simulink model "image_view"  (Simulink 7.8)
settings: Solver=ode45  StartTime=0.0  StopTime=30.0  RelTol=1e-3
undefined symbols (not defined in the file): gray, none, videoinput
libraries: imaqlib x1, visionsinks x1
settings Model: Creator=wildcat  LastModifiedBy=wildcat

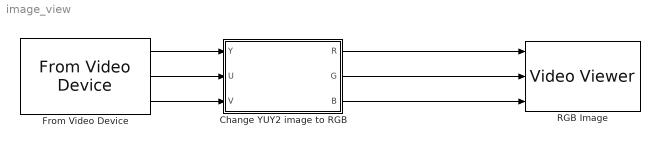
== system image_view ==
  Change YUY2 image to RGB : MATLAB Function  TreatAsAtomicUnit=on
  From Video Device : imaqlib/From Video Device  DeviceMenu=winvideo 1 (Microsoft LifeCam HD-3000)  Device=winvideo 1 (Microsoft LifeCam HD-3000)  ObjConstructor=videoinput('winvideo', 1)  VideoFormatMenu=YUY2_1280x720  VideoFormat=YUY2_1280x720  VideoSource=input1  ROIPosition=[0 0 720 1280]  EnableHWTrigger=off  TriggerConfiguration=none/none  SampleTime=1/30  OutputPortsMode=Separate color signals  DataType=uint8  CanDoHWTrigger=no  ReturnedColorSpace=YCbCr  BlockHandle=55.0015  ROIWidth=1280  ROIHeight=720  ROIColumn=0  ROIRow=0  EngXMLPath=C:\Program Files\MatlabR2011b\toolbox\imaq\imaq\private  DevXMLPath=C:\Program Files\MatlabR2011b\toolbox\imaq\imaqadaptors\win64  EngLibPath=C:\Program Files\MatlabR2011b\toolbox\imaq\imaqblks\imaqmex\win64
  RGB Image : visionsinks/Video Viewer  inputType=Obsolete7b  imagePorts=Separate color signals  useColorMap=off  colormapValue=gray(256)  specRange=off  minInputVal=0  maxInputVal=255  FigPos=[52 664 655 508]  AxisZoom=on  trueSizedOnce=off  OpenAtMdlStart=on
  wires:
  From Video Device/1 -> Change YUY2 image to RGB/1(Y)
  From Video Device/2 -> Change YUY2 image to RGB/2(U)
  From Video Device/3 -> Change YUY2 image to RGB/3(V)
  Change YUY2 image to RGB/3(B) -> RGB Image/3
  Change YUY2 image to RGB/2(G) -> RGB Image/2
  Change YUY2 image to RGB/1(R) -> RGB Image/1

== matlab function Change YUY2 image to RGB ==
  data: Y input double; R output double; G output double; B output double; U input double; V input double
function [R,G,B] = YUY2toRGB(Y,U,V)
%% input is (:,:,1:3), where
%% (:,:,1) is Y, (:,:,2) is U, (:,:,3) is V


%Y = single(data(:,:,1));
%U = single(data(:,:,2));
%V = single(data(:,:,3));

B = 1.164*(Y - 16) + 2.018*(U - 128);

G = 1.164*(Y - 16) - 0.813*(V - 128) - 0.391*(U - 128);

R = 1.164*(Y - 16) + 1.596*(V - 128);

R=uint8(R);
G=uint8(G);
B=uint8(B);
